simulink model "RF-simulink"  (R2019a)
settings: Solver=FixedStepAuto  StartTime=0.0  StopTime=10.0  RelTol=1e-3  EnableMultiTasking=on
undefined symbols (not defined in the file): CR, serial
libraries: instrumentlib x2
settings Model: ExtModeTrigDuration=2  Creator=Aster  LastModifiedBy=Aster
settings SolverCC: PositivePriorityOrder=on
settings OptimizationCC: EnhancedBackFolding=on  PassReuseOutputArgsAs=Individual arguments  MaxStackSize=64  OptimizeBlockOrder=speed  DifferentSizesBufferReuse=on  OptimizationCustomize=off
settings DebuggingCC: ParameterTunabilityLossMsg=error
settings HardwareCC: ProdBitPerInt=16  ProdBitPerPointer=16  ProdBitPerSizeT=16  ProdBitPerPtrDiffT=16  ProdLargestAtomicFloat=None  ProdWordSize=8  ProdHWDeviceType=Atmel->AVR  UseEmbeddedCoderFeatures=off  UseSimulinkCoderFeatures=off
settings SFSimCC: MATLABDynamicMemAlloc=off
settings RTWCC: SystemTargetFile=ert.tlc  HardwareBoard=Arduino Uno  TLCOptions=-aInlineSetEventsForThisBaseRateFcn=TLC_FALSE -aSuppressMultiTaskScheduler=TLC_FALSE -aRateBasedStepFcn=1  TemplateMakefile=ert_default_tmf  GenerateReport=on  Toolchain=Arduino AVR  BuildConfiguration=Faster Runs  IncludeHyperlinkInReport=on  LaunchReport=on  GenerateTraceInfo=on  GenerateTraceReport=on  GenerateTraceReportSl=on  GenerateTraceReportSf=on  GenerateTraceReportEml=on
settings CodeAppCC: ForceParamTrailComments=on  IgnoreCustomStorageClasses=off  OperatorAnnotations=on  SimulinkDataObjDesc=on  SFDataObjDesc=on  InsertBlockDesc=on
settings ERTTargetCC: SupportContinuousTime=on  SupportNonInlinedSFcns=on  SupportVariableSizeSignals=on  ExtModeStaticAllocSize=250

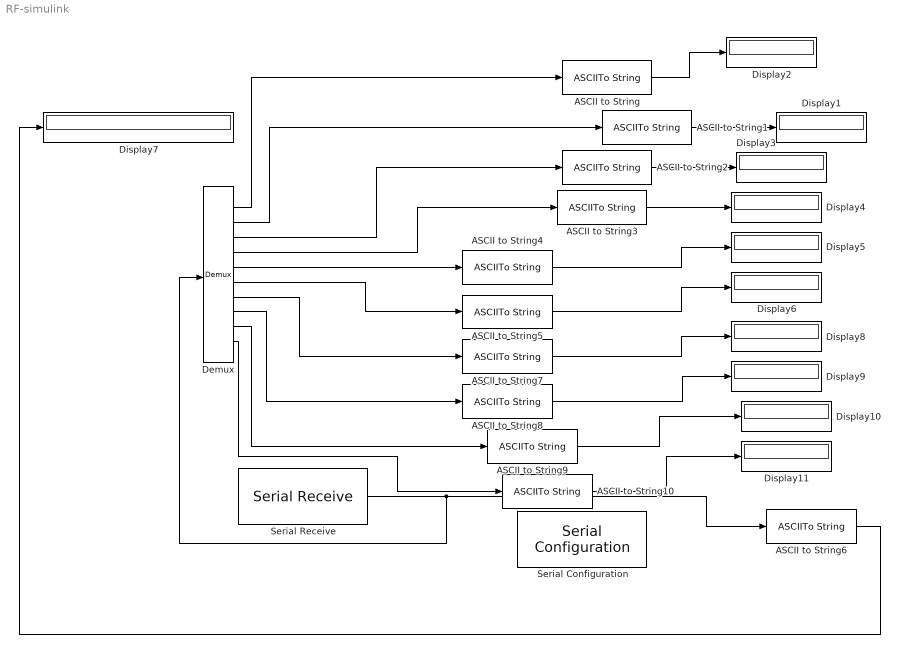
== system RF-simulink ==
  ASCII to String{,1..10} (11 alike) : ASCIIToString
  Demux : Demux  Outputs=10
  Display{1..11} (11 alike) : Display
      Display2 settings: Format=short_e
  Serial Configuration : instrumentlib/Serial Configuration  Priority=-200000  ComPortMenu=<Please select a port...>  ComPort=COM5  ObjConstructor=serial('COM5');  BaudRate=115200  DataBits=8  Parity=none  StopBits=1  FlowControl=hardware  Timeout=10  ByteOrder=LittleEndian
  Serial Receive : instrumentlib/Serial Receive  ComPortMenu=<Please select a port...>  ComPort=COM5  ObjConstructor=serial('COM5');  Terminator=CR ('\r')  DataSize="[1  13]"  DataType=uint8  EnableBlockingMode=on  ActionDataUnavailable=Error  CustomValue=33  SampleTime=0.01
  wires:
  Serial Receive/1 -> ASCII to String6/1, Demux/1
  Demux/2 -> ASCII to String1/1
  Demux/3 -> ASCII to String2/1
  Demux/4 -> ASCII to String3/1
  Demux/5 -> ASCII to String4/1
  Demux/1 -> ASCII to String/1
  ASCII to String/1 -> Display2/1
  ASCII to String1/1 -> Display1/1
  ASCII to String2/1 -> Display3/1
  ASCII to String3/1 -> Display4/1
  ASCII to String4/1 -> Display5/1
  Demux/6 -> ASCII to String5/1
  ASCII to String5/1 -> Display6/1
  ASCII to String6/1 -> Display7/1
  ASCII to String7/1 -> Display8/1
  Demux/7 -> ASCII to String7/1
  ASCII to String8/1 -> Display9/1
  ASCII to String9/1 -> Display10/1
  Demux/8 -> ASCII to String8/1
  Demux/9 -> ASCII to String9/1
  ASCII to String10/1 -> Display11/1
  Demux/10 -> ASCII to String10/1
